simulink model "Mooventure2016_Rev5"  (Simulink 7.7)
settings: Solver=FixedStepDiscrete  StartTime=0.0  StopTime=10  RelTol=1e-3
PreLoadFcn:
  | try, eval([bdroot '_setup']); catch, eval('model_setup', ''); end
InitFcn:
  | try, eval([bdroot '_setup']); catch, eval('model_setup', ''); end
undefined symbols (not defined in the file): ECM, H1, motohawk_build_version, motohawk_trunc_name, motohawk_vardec_config_group, motohawk_vardec_path, xD
libraries: MotoHawk_lib x976, motohawk_control_primitives_lib x41, simulink x27, motohawk_annotations_lib x3
(part 15 of 16)

== system Mooventure2016_Rev5/Foreground/Control/Hybrid Control Code/Cruise Control/Speed Resume ==
  In1 : Inport
  Detect Increase : simulink/Logic and Bit Operations/Detect Increase  SystemSampleTime=-1  vinit=0.0
  Enabled Subsystem1 : Subsystem  TreatAsAtomicUnit=on
  wires:
  In1/1 -> Detect Increase/1
  Detect Increase/1 -> Enabled Subsystem1/Enable

== system Mooventure2016_Rev5/Foreground/Control/Hybrid Control Code/Cruise Control/System Start ==
  In1 : Inport
  Enable : EnablePort
  Constant : Constant  OutDataTypeStr=boolean
  motohawk_data_write : MotoHawk_lib/Data Storage Blocks/motohawk_data_write  source=Lookup By Name  structure=Scalar  operation=Write entire data structure at once  sz_vec=9  sz_row=2  sz_col=9  typ=double  nam='CruiseSpeed'  checkNull=on  write_read_only=off  struct_inst_name=''  struct_name='MyStruct'
  motohawk_data_write1 : MotoHawk_lib/Data Storage Blocks/motohawk_data_write  source=Lookup By Name  structure=Scalar  operation=Write entire data structure at once  sz_vec=9  sz_row=2  sz_col=9  typ=boolean  nam='CruiseOn'  checkNull=on  write_read_only=off  struct_inst_name=''  struct_name='MyStruct'
  wires:
  In1/1 -> motohawk_data_write/1
  Constant/1 -> motohawk_data_write1/1

== system Mooventure2016_Rev5/Foreground/Control/Hybrid Control Code/Hybrid state limits1/Embedded MATLAB Function ==
  ecoMode_Enable : Inport
  SOC : Inport  Port=2
  CHESoC : Inport  Port=3
  SMESoC : Inport  Port=4
  nEV : Inport  Port=5
  Embedded MATLAB Function : Stateflow chart  TreatAsAtomicUnit=on
  state : Outport
  wires:
  ecoMode_Enable/1 -> Embedded MATLAB Function/1(ecoMode_Enable)
  SOC/1 -> Embedded MATLAB Function/2(SOC)
  CHESoC/1 -> Embedded MATLAB Function/3(CHESoC)
  SMESoC/1 -> Embedded MATLAB Function/4(SMESoC)
  nEV/1 -> Embedded MATLAB Function/5(nEV)
  Embedded MATLAB Function/1(state) -> state/1  "state"

== system Mooventure2016_Rev5/Foreground/Control/Hybrid Control Code/IPT/CurrentLimiting_TurboRequest ==
  BatteryCurrent : Inport
  First Order Low Pass (Tunable) : Subsystem  mask(First-Order Low-Pass Filter (Tunable)){nam='Overcurrent_Tq_Lim_Filter', samp_time=-1, group=motohawk_vardec_path(gcb)}
      mask prompts: nam "Name"; samp_time "Sample Time"; group "MotoTune Group String"
      mask help:
      | Discrete first-order low-pass filter, with calibratable time-constant.
      |
      | If 'Sample Time' is -1, then extra code and RAM will be generated to dynamically calculate dt.
      mask Display:
      | patch([0 0 1 1], [0 0.075 0.075 0], [230/255 0/255 0/255])
      | patch([0 0 1 1], [0.025 0.05 0.05 0.025], [150/255 0/255 0/255])
      | patch([0 0 1 1], [0 0.025 0.025 0], [0/255 0/255 0/255])
      | 
      | disp('1st-Order\nLow Pass');
  Gain : Gain  Gain=-1
  OvercurrentIntegralGenerator : Subsystem
  motohawk_probe : MotoHawk_lib/Calibration & Probing Blocks/motohawk_probe  nam='overcurrentintegral_prb'  show_more=off  name_source=Use Parameter  read_level=1  view_as=Number  enum_struct={'Disabled', 'Enabled'}  vector_style=Wide Row  use_help_units=off  help=''  units=''  use_header_enum=off  row_header_enum={}  col_header_enum={}  use_precision=off  precision=''  gain=1  offset=0  exp=1  use_mototune_group=off  mototune_group=motohawk_vardec_path(gcb)
  motohawk_probe1 : MotoHawk_lib/Calibration & Probing Blocks/motohawk_probe  nam='Overcurrent_Torque_Derate_prb'  show_more=off  name_source=Use Parameter  read_level=1  view_as=Number  enum_struct={'Disabled', 'Enabled'}  vector_style=Wide Row  use_help_units=off  help=''  units=''  use_header_enum=off  row_header_enum={}  col_header_enum={}  use_precision=off  precision=''  gain=1  offset=0  exp=1  use_mototune_group=off  mototune_group=motohawk_vardec_path(gcb)
  motohawk_table_1d : MotoHawk_lib/Lookup Tables/motohawk_table_1d  SystemSampleTime=-1  nam='TorqueLimMultiplier'  bp_nam='ModifiedAmpSec'  breakpoint_data=[0,200,900,1500]  table_data=[1,1,0,0]  show_more=off  bp_data_type=Inherit from 'Breakpoint Data'  bp_storage=Constant  table_data_type=Inherit from 'Table Data'  storage=NonAdaptive  read_level=1  write_level=1  ovr_cals=on  use_help=off  help=''  bp_units=''  table_units=''  use_min_max=off  bp_min_val=-inf  bp_max_val=inf  min_val=-inf  max_val=inf  use_precision=off  use_breakpoint=off  b_precision=''  b_gain=1  b_offset=0  b_exp=1  use_table=off  t_precision=''  t_gain=1  t_offset=0  t_exp=1  use_links=off  input_name=''  output_name=''  use_mototune_group=off  mototune_group=motohawk_vardec_path(gcb)
  TorqueMultiplier : Outport
  wires:
  OvercurrentIntegralGenerator/1(OverCurrentIntegral) -> motohawk_table_1d/1, motohawk_probe/1
  BatteryCurrent/1 -> Gain/1
  motohawk_table_1d/1 -> First Order Low Pass (Tunable)/1(in)
  Gain/1 -> OvercurrentIntegralGenerator/1(Current)
  First Order Low Pass (Tunable)/1(out) -> TorqueMultiplier/1, motohawk_probe1/1

== system Mooventure2016_Rev5/Foreground/Control/Hybrid Control Code/IPT/Drive ==
  Enable : EnablePort
  Constant1 : Constant
  motohawk_override_abs4 : MotoHawk_lib/Calibration & Probing Blocks/motohawk_override_abs  SystemSampleTime=-1  parent_name='Torque_Reverse_Override'  parent_val=1  show_more=on  name_source=Use Parameter  parent_read_level=1  parent_override_level=1  view_as=Number  enum_struct={'Disabled', 'Enabled'}  use_help_units=off  parent_help=''  parent_units=''  use_min_max=on  parent_min=-inf  parent_max=inf  use_precision=off  parent_precision=''  parent_gain=1  parent_offset=0  parent_exp=1  use_mototune_group=off  parent_group=motohawk_vardec_path(gcb)
  IPT_Torque : Outport  OutputWhenDisabled=reset  InitialOutput=[0]
  wires:
  Constant1/1 -> motohawk_override_abs4/1
  motohawk_override_abs4/1 -> IPT_Torque/1

== system Mooventure2016_Rev5/Foreground/Control/Hybrid Control Code/IPT/First Order Low Pass (Tunable) ==
  note: Tunable 1st-Order Low-Pass Filter
  in : Inport
  First Order Low Pass : motohawk_control_primitives_lib/First Order Low Pass  SystemSampleTime=-1
  MinMax : MinMax  Function=max  Inputs=2  SaturateOnIntegerOverflow=on  InputSameDT=on
  Product : Product  Inputs=*/  SaturateOnIntegerOverflow=on  InputSameDT=on  OutDataTypeStr=Inherit: Same as first input
  motohawk_calibration : MotoHawk_lib/Calibration & Probing Blocks/motohawk_calibration  nam=nam  val=.4  storage=Calibration  show_more=on  name_source=Use Parameter  data_type=Inherit from 'Default Value'  read_level=1  write_level=1  ovr_cals=on  view_as=Number  enum_struct={'Disabled', 'Enabled'}  vector_style=Wide Row  use_help_units=on  help='Filter time constant'  units='sec'  use_header_enum=off  row_header_enum={}  col_header_enum={}  use_min_max=off  min_val=-inf  max_val=inf  use_precision=off  precision=''  gain=1  offset=0  exp=1  use_mototune_group=on  mototune_group=group %% motohawk_vardec_config_group(group)
  motohawk_delta_time : MotoHawk_lib/Extra Development Blocks/motohawk_delta_time  samp_time=samp_time  init_val=0  mode=Seconds (double)
  out : Outport
  wires:
  First Order Low Pass/1 -> out/1
  in/1 -> First Order Low Pass/1
  motohawk_delta_time/1 -> Product/1, MinMax/1
  Product/1 -> First Order Low Pass/2
  MinMax/1 -> Product/2
  motohawk_calibration/1 -> MinMax/2

== system Mooventure2016_Rev5/Foreground/Control/Hybrid Control Code/IPT/Neutral ==
  Enable : EnablePort
  Constant : Constant  Value=0
  IPT_Torque : Outport
  wires:
  Constant/1 -> IPT_Torque/1  "IPT_Torque"

== system Mooventure2016_Rev5/Foreground/Control/Hybrid Control Code/IPT/Reverse ==
  Enable : EnablePort
  Constant1 : Constant  Value=-1
  motohawk_override_abs4 : MotoHawk_lib/Calibration & Probing Blocks/motohawk_override_abs  SystemSampleTime=-1  parent_name='Torque_Reverse_Override69'  parent_val=1  show_more=on  name_source=Use Parameter  parent_read_level=1  parent_override_level=1  view_as=Number  enum_struct={'Disabled', 'Enabled'}  use_help_units=off  parent_help=''  parent_units=''  use_min_max=on  parent_min=-inf  parent_max=inf  use_precision=off  parent_precision=''  parent_gain=1  parent_offset=0  parent_exp=1  use_mototune_group=off  parent_group=motohawk_vardec_path(gcb)
  IPT_Torque : Outport  OutputWhenDisabled=reset  InitialOutput=[0]
  wires:
  Constant1/1 -> motohawk_override_abs4/1
  motohawk_override_abs4/1 -> IPT_Torque/1

== system Mooventure2016_Rev5/Foreground/Inputs/Analog Inputs/Coolant/Heater Core Low Pass ==
  note: Tunable 1st-Order Low-Pass Filter
  in : Inport
  First Order Low Pass : motohawk_control_primitives_lib/First Order Low Pass  SystemSampleTime=-1
  MinMax : MinMax  Function=max  Inputs=2  SaturateOnIntegerOverflow=on  InputSameDT=on
  Product : Product  Inputs=*/  SaturateOnIntegerOverflow=on  InputSameDT=on  OutDataTypeStr=Inherit: Same as first input
  motohawk_calibration : MotoHawk_lib/Calibration & Probing Blocks/motohawk_calibration  nam=nam  val=.4  storage=Calibration  show_more=on  name_source=Use Parameter  data_type=Inherit from 'Default Value'  read_level=1  write_level=1  ovr_cals=on  view_as=Number  enum_struct={'Disabled', 'Enabled'}  vector_style=Wide Row  use_help_units=on  help='Filter time constant'  units='sec'  use_header_enum=off  row_header_enum={}  col_header_enum={}  use_min_max=off  min_val=-inf  max_val=inf  use_precision=off  precision=''  gain=1  offset=0  exp=1  use_mototune_group=on  mototune_group=group %% motohawk_vardec_config_group(group)
  motohawk_delta_time : MotoHawk_lib/Extra Development Blocks/motohawk_delta_time  samp_time=samp_time  init_val=0  mode=Seconds (double)
  out : Outport
  wires:
  First Order Low Pass/1 -> out/1
  in/1 -> First Order Low Pass/1
  motohawk_delta_time/1 -> Product/1, MinMax/1
  Product/1 -> First Order Low Pass/2
  MinMax/1 -> Product/2
  motohawk_calibration/1 -> MinMax/2

== system Mooventure2016_Rev5/Foreground/Inputs/Analog Inputs/Coolant/Radiator Low Pass ==
  note: Tunable 1st-Order Low-Pass Filter
  in : Inport
  First Order Low Pass : motohawk_control_primitives_lib/First Order Low Pass  SystemSampleTime=-1
  MinMax : MinMax  Function=max  Inputs=2  SaturateOnIntegerOverflow=on  InputSameDT=on
  Product : Product  Inputs=*/  SaturateOnIntegerOverflow=on  InputSameDT=on  OutDataTypeStr=Inherit: Same as first input
  motohawk_calibration : MotoHawk_lib/Calibration & Probing Blocks/motohawk_calibration  nam=nam  val=.4  storage=Calibration  show_more=on  name_source=Use Parameter  data_type=Inherit from 'Default Value'  read_level=1  write_level=1  ovr_cals=on  view_as=Number  enum_struct={'Disabled', 'Enabled'}  vector_style=Wide Row  use_help_units=on  help='Filter time constant'  units='sec'  use_header_enum=off  row_header_enum={}  col_header_enum={}  use_min_max=off  min_val=-inf  max_val=inf  use_precision=off  precision=''  gain=1  offset=0  exp=1  use_mototune_group=on  mototune_group=group %% motohawk_vardec_config_group(group)
  motohawk_delta_time : MotoHawk_lib/Extra Development Blocks/motohawk_delta_time  samp_time=samp_time  init_val=0  mode=Seconds (double)
  out : Outport
  wires:
  First Order Low Pass/1 -> out/1
  in/1 -> First Order Low Pass/1
  motohawk_delta_time/1 -> Product/1, MinMax/1
  Product/1 -> First Order Low Pass/2
  MinMax/1 -> Product/2
  motohawk_calibration/1 -> MinMax/2

== system Mooventure2016_Rev5/Foreground/Inputs/Battery_Inputs/SOC Filter/First Order Low Pass (Tunable) ==
  note: Tunable 1st-Order Low-Pass Filter
  in : Inport
  First Order Low Pass : motohawk_control_primitives_lib/First Order Low Pass  SystemSampleTime=-1
  MinMax : MinMax  Function=max  Inputs=2  SaturateOnIntegerOverflow=on  InputSameDT=on
  Product : Product  Inputs=*/  SaturateOnIntegerOverflow=on  InputSameDT=on  OutDataTypeStr=Inherit: Same as first input
  motohawk_calibration : MotoHawk_lib/Calibration & Probing Blocks/motohawk_calibration  nam=nam  val=5  storage=Calibration  show_more=on  name_source=Use Parameter  data_type=Inherit from 'Default Value'  read_level=1  write_level=1  ovr_cals=on  view_as=Number  enum_struct={'Disabled', 'Enabled'}  vector_style=Wide Row  use_help_units=on  help='Filter time constant'  units='sec'  use_header_enum=off  row_header_enum={}  col_header_enum={}  use_min_max=off  min_val=-inf  max_val=inf  use_precision=off  precision=''  gain=1  offset=0  exp=1  use_mototune_group=on  mototune_group=group %% motohawk_vardec_config_group(group)
  motohawk_delta_time : MotoHawk_lib/Extra Development Blocks/motohawk_delta_time  samp_time=samp_time  init_val=0  mode=Seconds (double)
  out : Outport
  wires:
  First Order Low Pass/1 -> out/1
  in/1 -> First Order Low Pass/1
  motohawk_delta_time/1 -> Product/1, MinMax/1
  Product/1 -> First Order Low Pass/2
  MinMax/1 -> Product/2
  motohawk_calibration/1 -> MinMax/2

== system Mooventure2016_Rev5/Foreground/Inputs/Battery_Inputs/Voltage Filter/First Order Low Pass (Tunable) ==
  note: Tunable 1st-Order Low-Pass Filter
  in : Inport
  First Order Low Pass : motohawk_control_primitives_lib/First Order Low Pass  SystemSampleTime=-1
  MinMax : MinMax  Function=max  Inputs=2  SaturateOnIntegerOverflow=on  InputSameDT=on
  Product : Product  Inputs=*/  SaturateOnIntegerOverflow=on  InputSameDT=on  OutDataTypeStr=Inherit: Same as first input
  motohawk_calibration : MotoHawk_lib/Calibration & Probing Blocks/motohawk_calibration  nam=nam  val=5  storage=Calibration  show_more=on  name_source=Use Parameter  data_type=Inherit from 'Default Value'  read_level=1  write_level=1  ovr_cals=on  view_as=Number  enum_struct={'Disabled', 'Enabled'}  vector_style=Wide Row  use_help_units=on  help='Filter time constant'  units='sec'  use_header_enum=off  row_header_enum={}  col_header_enum={}  use_min_max=off  min_val=-inf  max_val=inf  use_precision=off  precision=''  gain=1  offset=0  exp=1  use_mototune_group=on  mototune_group=group %% motohawk_vardec_config_group(group)
  motohawk_delta_time : MotoHawk_lib/Extra Development Blocks/motohawk_delta_time  samp_time=samp_time  init_val=0  mode=Seconds (double)
  out : Outport
  wires:
  First Order Low Pass/1 -> out/1
  in/1 -> First Order Low Pass/1
  motohawk_delta_time/1 -> Product/1, MinMax/1
  Product/1 -> First Order Low Pass/2
  MinMax/1 -> Product/2
  motohawk_calibration/1 -> MinMax/2

== system Mooventure2016_Rev5/Foreground/Control/Faults/Accesories/HV-Heater System/Triggered Subsystem ==
  In1 : Inport
  Trigger : TriggerPort
  motohawk_data_write : MotoHawk_lib/Data Storage Blocks/motohawk_data_write  source=Lookup By Name  structure=Scalar  operation=Write entire data structure at once  sz_vec=9  sz_row=2  sz_col=9  typ=double  nam='TempReading'  checkNull=on  write_read_only=off  struct_inst_name=''  struct_name='MyStruct'
  wires:
  In1/1 -> motohawk_data_write/1

== system Mooventure2016_Rev5/Foreground/Control/Hybrid Control Code/Cruise Control/Speed Changing/Speed Decrease ==
  Enable : EnablePort
  Add : Sum  Inputs=+-
  Constant : Constant
  motohawk_data_read1 : MotoHawk_lib/Data Storage Blocks/motohawk_data_read  source=Lookup By Name  structure=Scalar  operation=Read scalar from location by index  sz_vec=4  sz_row=2  sz_col=3  typ=double  nam='CruiseSpeed'  checkNull=on  struct_inst_name='MyData'  struct_nam='MyStruct'
  motohawk_data_write : MotoHawk_lib/Data Storage Blocks/motohawk_data_write  source=Lookup By Name  structure=Scalar  operation=Write entire data structure at once  sz_vec=9  sz_row=2  sz_col=9  typ=double  nam='CruiseSpeed'  checkNull=on  write_read_only=off  struct_inst_name=''  struct_name='MyStruct'
  wires:
  motohawk_data_read1/1 -> Add/1
  Constant/1 -> Add/2
  Add/1 -> motohawk_data_write/1

== system Mooventure2016_Rev5/Foreground/Control/Hybrid Control Code/Cruise Control/Speed Changing/Speed Increase ==
  Enable : EnablePort
  Add : Sum
  Constant : Constant
  motohawk_data_read1 : MotoHawk_lib/Data Storage Blocks/motohawk_data_read  source=Lookup By Name  structure=Scalar  operation=Read scalar from location by index  sz_vec=4  sz_row=2  sz_col=3  typ=double  nam='CruiseSpeed'  checkNull=on  struct_inst_name='MyData'  struct_nam='MyStruct'
  motohawk_data_write : MotoHawk_lib/Data Storage Blocks/motohawk_data_write  source=Lookup By Name  structure=Scalar  operation=Write entire data structure at once  sz_vec=9  sz_row=2  sz_col=9  typ=double  nam='CruiseSpeed'  checkNull=on  write_read_only=off  struct_inst_name=''  struct_name='MyStruct'
  wires:
  motohawk_data_read1/1 -> Add/1
  Constant/1 -> Add/2
  Add/1 -> motohawk_data_write/1

== system Mooventure2016_Rev5/Foreground/Control/Hybrid Control Code/Cruise Control/Speed Control/PID With Damper Terms (Tunable) ==
  note: PID With Damper Terms
      | With Calibratable Parameters and Observable States
  Actual : Inport
  SetPoint : Inport  Port=2
  ResetITerm : Inport  Port=3
  Ground2 : Ground
  PID With Damper Terms : Subsystem  Description=|  AncestorBlock=motohawk_control_primitives_lib/PID With Damper Terms  mask(PID with Damper Terms){samp_time=SampleTime}
      | /* Name: ErrorGain Unit:mult ClassID:VAR StorageID:FLASH Access:RW4+RW3+NA2+NA1 TypeID:UINT4                   
      |    Gain:0.000000001 Min:0.000000000 Max:4.000000000 Format:10.9 UpdateID:REMOTE Help:"This gain is applied to "
      |    "the error term before it is used to calculate the P, I and D terms." VardecSig:6C */                       
      |                                                                                                                
      | /* Name: ITermLowerLim Unit:0 ClassID:VAR StorageID:FLASH Access:RW4+RW3+NA2+NA1 TypeID:SINT2 Gain:0.1         
      |    Min:-3276.8 Max:3276.7 Format:5.1 UpdateID:REMOTE Help:"Lower limit on the I-term value." VardecSig:6C */   
      |                                                                                                                
      | /* Name: ITermUpperLim ClassID:VAR StorageID:FLASH Access:RW4+RW3+NA2+NA1 TypeID:SINT2 Gain:0.1 Min:-3276.8    
      |    Max:3276.7 Format:5.1 UpdateID:REMOTE Help:"Upper limit on I-term value." VardecSig:6C */                   
      |                                                                                                                
      | /* Name: PIDOutLowerLim ClassID:VAR StorageID:FLASH Access:RW4+RW3+NA2+NA1 TypeID:SINT2 Gain:0.1               
      |    Min:-3276.8 Max:3276.7 Format:5.1 UpdateID:REMOTE Help:"Lower limit on PID output." VardecSig:6C */         
      |                                                                                                                
      | /* Name: PIDOutUpperLim ClassID:VAR StorageID:FLASH Access:RW4+RW3+NA2+NA1 TypeID:SINT2 Gain:0.1               
      |    Min:-3276.8 Max:3276.7 Format:3.1 UpdateID:REMOTE Help:"Upper limit on PID output." VardecSig:6C */         
      |                                                                                                                
      | /* Name: PIDError ClassID:VAR StorageID:RAM Access:RO4+RO3+NA2+NA1 TypeID:SINT2 Gain:1 Min:-32768.00           
      |    Max:32767.00 Format:4.2 UpdateID:BACKGND Help:"Current controller error input value." VardecSig:6C */       
      |                                                                                                                
      | /* Name: PTerm ClassID:VAR StorageID:RAM Access:RO4+RO3+NA2+NA1 TypeID:SINT2 Gain:1 Min:-32768.00              
      |    Max:32767.00 Format:4.2 UpdateID:BACKGND Help:"Current P-term value" VardecSig:6C */                        
      |                                                                                                                
      | /* Name: ITerm ClassID:VAR StorageID:RAM Access:RO4+RO3+NA2+NA1 TypeID:SINT2 Gain:1 Min:-32768.00              
      |    Max:32767.00 Format:4.2 UpdateID:BACKGND Help:"Current I-term value" VardecSig:6C */                        
      |                                                                                                                
      | /* Name: DTerm ClassID:VAR StorageID:RAM Access:RO4+RO3+NA2+NA1 TypeID:SINT2 Gain:1 Min:-32768.00              
      |    Max:32767.00 Format:4.2 UpdateID:BACKGND Help:"Current D-term value" VardecSig:6C */                        
      |                                                                                                                
      | /* Name: DamperTerm ClassID:VAR StorageID:RAM Access:RO4+RO3+NA2+NA1 TypeID:SINT2 Gain:1 Min:-32768.00         
      |    Max:32767.00 Format:4.2 UpdateID:BACKGND Help:"Current Damper-term value" VardecSig:6C */                   
      |                                                                                                                
      | /* Name: PIDOutput ClassID:VAR StorageID:FLASH Access:RW4+RW3+NA2+NA1 TypeID:SINT2 Gain:1 Min:-32768.00        
      |    Max:32767.00 Format:4.2 UpdateID:REMOTE Help:"PID current output." VardecSig:6C */
      mask prompts: samp_time "Sample Time"
      mask help:
      | Resettable PID controller with damper terms and limits on the I-term.
      |
      | If 'Sample Time' is -1, then extra code and RAM will be generated to dynamically calculate dt.
      mask Display:
      | patch([0 0 1 1], 0.5*[0 0.075 0.075 0], [230/255 0/255 0/255])
      | patch([0 0 1 1], 0.5*[0.025 0.05 0.05 0.025], [150/255 0/255 0/255])
      | patch([0 0 1 1], 0.5*[0 0.025 0.025 0], [0/255 0/255 0/255])
      | 
      | disp('\fontsize{16}\bf\itPIDD', 'texmode', 'on')
  Saturation (Tunable) : motohawk_control_primitives_lib/Saturation (Tunable)  SystemSampleTime=-1  prefix=prefix  units=units  grp=grp
  Sum : Sum  Inputs=++|  InputSameDT=on
  motohawk_calibration : MotoHawk_lib/Calibration & Probing Blocks/motohawk_calibration  nam=[prefix 'PGain']  val=1  storage=Calibration  show_more=on  name_source=Use Parameter  data_type=Inherit from 'Default Value'  read_level=1  write_level=1  ovr_cals=on  view_as=Number  enum_struct={'Disabled', 'Enabled'}  vector_style=Wide Row  use_help_units=on  help='PID Proportional Gain'  units='mult'  use_header_enum=off  row_header_enum={}  col_header_enum={}  use_min_max=off  min_val=-inf  max_val=inf  use_precision=off  precision=''  gain=1  offset=0  exp=1  use_mototune_group=on  mototune_group=grp
  motohawk_calibration1 : MotoHawk_lib/Calibration & Probing Blocks/motohawk_calibration  nam=[prefix 'DGain']  val=1  storage=Calibration  show_more=on  name_source=Use Parameter  data_type=Inherit from 'Default Value'  read_level=1  write_level=1  ovr_cals=on  view_as=Number  enum_struct={'Disabled', 'Enabled'}  vector_style=Wide Row  use_help_units=on  help='PID Derivative Gain'  units='mult'  use_header_enum=off  row_header_enum={}  col_header_enum={}  use_min_max=off  min_val=-inf  max_val=inf  use_precision=off  precision=''  gain=1  offset=0  exp=1  use_mototune_group=on  mototune_group=grp
  motohawk_calibration2 : MotoHawk_lib/Calibration & Probing Blocks/motohawk_calibration  nam=[prefix 'IGain']  val=1  storage=Calibration  show_more=on  name_source=Use Parameter  data_type=Inherit from 'Default Value'  read_level=1  write_level=1  ovr_cals=on  view_as=Number  enum_struct={'Disabled', 'Enabled'}  vector_style=Wide Row  use_help_units=on  help='PID Integral Gain'  units='mult'  use_header_enum=off  row_header_enum={}  col_header_enum={}  use_min_max=off  min_val=-inf  max_val=inf  use_precision=off  precision=''  gain=1  offset=0  exp=1  use_mototune_group=on  mototune_group=grp
  motohawk_calibration3 : MotoHawk_lib/Calibration & Probing Blocks/motohawk_calibration  nam=[prefix 'IMin']  val=0  storage=Calibration  show_more=on  name_source=Use Parameter  data_type=Inherit from 'Default Value'  read_level=1  write_level=1  ovr_cals=on  view_as=Number  enum_struct={'Disabled', 'Enabled'}  vector_style=Wide Row  use_help_units=on  help='PID Integrator Lower Limit'  units=units  use_header_enum=off  row_header_enum={}  col_header_enum={}  use_min_max=off  min_val=-inf  max_val=inf  use_precision=off  precision=''  gain=1  offset=0  exp=1  use_mototune_group=on  mototune_group=grp
  motohawk_calibration4 : MotoHawk_lib/Calibration & Probing Blocks/motohawk_calibration  nam=[prefix 'IMax']  val=1  storage=Calibration  show_more=on  name_source=Use Parameter  data_type=Inherit from 'Default Value'  read_level=1  write_level=1  ovr_cals=on  view_as=Number  enum_struct={'Disabled', 'Enabled'}  vector_style=Wide Row  use_help_units=on  help='PID Integrator Upper Limit'  units=units  use_header_enum=off  row_header_enum={}  col_header_enum={}  use_min_max=off  min_val=-inf  max_val=inf  use_precision=off  precision=''  gain=1  offset=0  exp=1  use_mototune_group=on  mototune_group=grp
  motohawk_calibration5 : MotoHawk_lib/Calibration & Probing Blocks/motohawk_calibration  nam=[prefix 'DCOffset']  val=0  storage=Calibration  show_more=on  name_source=Use Parameter  data_type=Inherit from 'Default Value'  read_level=1  write_level=1  ovr_cals=on  view_as=Number  enum_struct={'Disabled', 'Enabled'}  vector_style=Wide Row  use_help_units=on  help='PID Output DC Offset'  units=units  use_header_enum=off  row_header_enum={}  col_header_enum={}  use_min_max=off  min_val=-inf  max_val=inf  use_precision=off  precision=''  gain=1  offset=0  exp=1  use_mototune_group=on  mototune_group=grp
  motohawk_calibration6 : MotoHawk_lib/Calibration & Probing Blocks/motohawk_calibration  nam=[prefix 'ErrorGain']  val=1  storage=Calibration  show_more=on  name_source=Use Parameter  data_type=Inherit from 'Default Value'  read_level=1  write_level=1  ovr_cals=on  view_as=Number  enum_struct={'Disabled', 'Enabled'}  vector_style=Wide Row  use_help_units=on  help='PID Error Gain'  units='mult'  use_header_enum=off  row_header_enum={}  col_header_enum={}  use_min_max=off  min_val=-inf  max_val=inf  use_precision=off  precision=''  gain=1  offset=0  exp=1  use_mototune_group=on  mototune_group=grp
  motohawk_calibration7 : MotoHawk_lib/Calibration & Probing Blocks/motohawk_calibration  nam=[prefix 'DampGainUp']  val=1  storage=Calibration  show_more=on  name_source=Use Parameter  data_type=Inherit from 'Default Value'  read_level=1  write_level=1  ovr_cals=on  view_as=Number  enum_struct={'Disabled', 'Enabled'}  vector_style=Wide Row  use_help_units=on  help='PID Damper Gain - Up Direction'  units='mult'  use_header_enum=off  row_header_enum={}  col_header_enum={}  use_min_max=off  min_val=-inf  max_val=inf  use_precision=off  precision=''  gain=1  offset=0  exp=1  use_mototune_group=on  mototune_group=grp
  motohawk_calibration8 : MotoHawk_lib/Calibration & Probing Blocks/motohawk_calibration  nam=[prefix 'DampGainDown']  val=1  storage=Calibration  show_more=on  name_source=Use Parameter  data_type=Inherit from 'Default Value'  read_level=1  write_level=1  ovr_cals=on  view_as=Number  enum_struct={'Disabled', 'Enabled'}  vector_style=Wide Row  use_help_units=on  help='PID Damper Gain - Down Direction'  units='mult'  use_header_enum=off  row_header_enum={}  col_header_enum={}  use_min_max=off  min_val=-inf  max_val=inf  use_precision=off  precision=''  gain=1  offset=0  exp=1  use_mototune_group=on  mototune_group=grp
  motohawk_probe : MotoHawk_lib/Calibration & Probing Blocks/motohawk_probe  nam=[prefix 'Out']  show_more=on  name_source=Use Parameter  read_level=1  view_as=Number  enum_struct={'Disabled', 'Enabled'}  vector_style=Wide Row  use_help_units=on  help='PID Final Output'  units=units  use_header_enum=off  row_header_enum={}  col_header_enum={}  use_precision=off  precision=''  gain=1  offset=0  exp=1  use_mototune_group=on  mototune_group=grp
  motohawk_probe1 : MotoHawk_lib/Calibration & Probing Blocks/motohawk_probe  nam=[prefix 'PTerm']  show_more=on  name_source=Use Parameter  read_level=1  view_as=Number  enum_struct={'Disabled', 'Enabled'}  vector_style=Wide Row  use_help_units=on  help='PID Proportional Term'  units=units  use_header_enum=off  row_header_enum={}  col_header_enum={}  use_precision=off  precision=''  gain=1  offset=0  exp=1  use_mototune_group=on  mototune_group=grp
  motohawk_probe2 : MotoHawk_lib/Calibration & Probing Blocks/motohawk_probe  nam=[prefix 'ITerm']  show_more=on  name_source=Use Parameter  read_level=1  view_as=Number  enum_struct={'Disabled', 'Enabled'}  vector_style=Wide Row  use_help_units=on  help='PID Integrator Term'  units=units  use_header_enum=off  row_header_enum={}  col_header_enum={}  use_precision=off  precision=''  gain=1  offset=0  exp=1  use_mototune_group=on  mototune_group=grp
  motohawk_probe3 : MotoHawk_lib/Calibration & Probing Blocks/motohawk_probe  nam=[prefix 'DTerm']  show_more=on  name_source=Use Parameter  read_level=1  view_as=Number  enum_struct={'Disabled', 'Enabled'}  vector_style=Wide Row  use_help_units=on  help='PID Derivative Term'  units=units  use_header_enum=off  row_header_enum={}  col_header_enum={}  use_precision=off  precision=''  gain=1  offset=0  exp=1  use_mototune_group=on  mototune_group=grp
  motohawk_probe4 : MotoHawk_lib/Calibration & Probing Blocks/motohawk_probe  nam=[prefix 'Error']  show_more=on  name_source=Use Parameter  read_level=1  view_as=Number  enum_struct={'Disabled', 'Enabled'}  vector_style=Wide Row  use_help_units=on  help='PID Error Term'  units=units  use_header_enum=off  row_header_enum={}  col_header_enum={}  use_precision=off  precision=''  gain=1  offset=0  exp=1  use_mototune_group=on  mototune_group=grp
  motohawk_probe5 : MotoHawk_lib/Calibration & Probing Blocks/motohawk_probe  nam=[prefix 'DampTerm']  show_more=on  name_source=Use Parameter  read_level=1  view_as=Number  enum_struct={'Disabled', 'Enabled'}  vector_style=Wide Row  use_help_units=on  help='PID Damper Term'  units=units  use_header_enum=off  row_header_enum={}  col_header_enum={}  use_precision=off  precision=''  gain=1  offset=0  exp=1  use_mototune_group=on  mototune_group=grp
  Out : Outport
  wires:
  motohawk_calibration5/1 -> Sum/1
  Sum/1 -> Saturation (Tunable)/1
  ResetITerm/1 -> PID With Damper Terms/12(I_reset)
  Ground2/1 -> PID With Damper Terms/9(IC)
  motohawk_calibration1/1 -> PID With Damper Terms/6(k_D)
  motohawk_calibration2/1 -> PID With Damper Terms/5(k_I)
  motohawk_calibration/1 -> PID With Damper Terms/4(k_P)
  PID With Damper Terms/3(P_term) -> motohawk_probe1/1
  Actual/1 -> PID With Damper Terms/1(Actual)
  SetPoint/1 -> PID With Damper Terms/2(SetPt)
  PID With Damper Terms/1(Out) -> Sum/2
  motohawk_calibration6/1 -> PID With Damper Terms/3(k_Err)
  motohawk_calibration3/1 -> PID With Damper Terms/10(I_min)
  motohawk_calibration4/1 -> PID With Damper Terms/11(I_max)
  PID With Damper Terms/4(I_term) -> motohawk_probe2/1
  PID With Damper Terms/5(D_term) -> motohawk_probe3/1
  PID With Damper Terms/2(Err) -> motohawk_probe4/1
  motohawk_calibration7/1 -> PID With Damper Terms/7(k_Dmp,u)
  motohawk_calibration8/1 -> PID With Damper Terms/8(k_Dmp,d)
  PID With Damper Terms/6(Dmp_term) -> motohawk_probe5/1
  Saturation (Tunable)/1 -> Out/1, motohawk_probe/1

== system Mooventure2016_Rev5/Foreground/Control/Hybrid Control Code/Cruise Control/Speed Resume/Enabled Subsystem1 ==
  Enable : EnablePort
  Constant : Constant  OutDataTypeStr=boolean
  motohawk_data_write1 : MotoHawk_lib/Data Storage Blocks/motohawk_data_write  source=Lookup By Name  structure=Scalar  operation=Write entire data structure at once  sz_vec=9  sz_row=2  sz_col=9  typ=boolean  nam='CruiseOn'  checkNull=on  write_read_only=off  struct_inst_name=''  struct_name='MyStruct'
  wires:
  Constant/1 -> motohawk_data_write1/1

== system Mooventure2016_Rev5/Foreground/Control/Hybrid Control Code/IPT/CurrentLimiting_TurboRequest/First Order Low Pass (Tunable) ==
  note: Tunable 1st-Order Low-Pass Filter
  in : Inport
  First Order Low Pass : motohawk_control_primitives_lib/First Order Low Pass  SystemSampleTime=-1
  MinMax : MinMax  Function=max  Inputs=2  SaturateOnIntegerOverflow=on  InputSameDT=on
  Product : Product  Inputs=*/  SaturateOnIntegerOverflow=on  InputSameDT=on  OutDataTypeStr=Inherit: Same as first input
  motohawk_calibration : MotoHawk_lib/Calibration & Probing Blocks/motohawk_calibration  nam=nam  val=.005  storage=Calibration  show_more=on  name_source=Use Parameter  data_type=Inherit from 'Default Value'  read_level=1  write_level=1  ovr_cals=on  view_as=Number  enum_struct={'Disabled', 'Enabled'}  vector_style=Wide Row  use_help_units=on  help='Filter time constant'  units='sec'  use_header_enum=off  row_header_enum={}  col_header_enum={}  use_min_max=off  min_val=-inf  max_val=inf  use_precision=off  precision=''  gain=1  offset=0  exp=1  use_mototune_group=on  mototune_group=group %% motohawk_vardec_config_group(group)
  motohawk_delta_time : MotoHawk_lib/Extra Development Blocks/motohawk_delta_time  samp_time=samp_time  init_val=0  mode=Seconds (double)
  out : Outport
  wires:
  First Order Low Pass/1 -> out/1
  in/1 -> First Order Low Pass/1
  motohawk_delta_time/1 -> Product/1, MinMax/1
  Product/1 -> First Order Low Pass/2
  MinMax/1 -> Product/2
  motohawk_calibration/1 -> MinMax/2

== system Mooventure2016_Rev5/Foreground/Control/Hybrid Control Code/IPT/CurrentLimiting_TurboRequest/OvercurrentIntegralGenerator ==
  note: max over current integral allowed
  Current : Inport
  Constant : Constant  Value=0
  Constant1 : Constant  Value=1500
  Constant2 : Constant  Value=0
  Constant3 : Constant  Value=0
  CurrentModifier : Subsystem
  Integrator : Subsystem  mask(Discrete Integrator){samp_time=-1}
      mask prompts: samp_time "Sample Time"
      mask help:
      | Resetable integrator with upper and lower windup limits.
      |
      | If 'Sample Time' is -1, then extra code and RAM will be generated to dynamically calculate dt.
      mask Display:
      | patch([0 0 1 1], 0.75*[0 0.075 0.075 0], [230/255 0/255 0/255])
      | patch([0 0 1 1], 0.75*[0.025 0.05 0.05 0.025], [150/255 0/255 0/255])
      | patch([0 0 1 1], 0.75*[0 0.025 0.025 0], [0/255 0/255 0/255])
      | 
      | disp('\fontsize{16}\bf\it\int dt', 'texmode', 'on')
  OverCurrentIntegral : Outport
  wires:
  Constant2/1 -> Integrator/3(IC)
  Constant/1 -> Integrator/4(Min)
  Constant1/1 -> Integrator/5(Max)
  Constant3/1 -> Integrator/2(Rst)
  CurrentModifier/1(Out1) -> Integrator/1(In)
  Current/1 -> CurrentModifier/1(In1)
  Integrator/1(Out) -> OverCurrentIntegral/1

== system Mooventure2016_Rev5/Foreground/Control/Hybrid Control Code/Cruise Control/Speed Control/PID With Damper Terms (Tunable)/PID With Damper Terms ==
  note: Universal PID Controller
      | with Dampers
  Actual : Inport
  SetPt : Inport  Port=2
  k_Err : Inport  Port=3
  k_P : Inport  Port=4
  k_I : Inport  Port=5
  k_D : Inport  Port=6
  k_Dmp,u : Inport  Port=7
  k_Dmp,d : Inport  Port=8
  IC : Inport  Port=9
  I_min : Inport  Port=10
  I_max : Inport  Port=11
  I_reset : Inport  Port=12
  Constant : Constant  Value=0  OutDataTypeStr=Inherit: Inherit via back propagation
  Data Type Conversion : DataTypeConversion  SaturateOnIntegerOverflow=on  RndMeth=Zero
  Derivitive1 : motohawk_control_primitives_lib/Derivitive  SystemSampleTime=-1  samp_time=samp_time
  Derivitive2 : motohawk_control_primitives_lib/Derivitive  SystemSampleTime=-1  samp_time=samp_time
  Derivitive3 : motohawk_control_primitives_lib/Derivitive  SystemSampleTime=-1  samp_time=samp_time
  Integrator : motohawk_control_primitives_lib/Integrator  SystemSampleTime=-1  samp_time=samp_time
  Product{1..5} (5 alike) : Product  InputSameDT=on  OutDataTypeStr=Inherit: Same as first input
  Relational Operator : RelationalOperator  Operator=>  ZeroCross=off  InputSameDT=on
  Sum : Sum  Inputs=-|+|+|+  SaturateOnIntegerOverflow=on  InputSameDT=on  OutDataTypeStr=Inherit: Same as first input
  Sum2 : Sum  Inputs=-|+  SaturateOnIntegerOverflow=on  InputSameDT=on  OutDataTypeStr=Inherit: Same as first input
  Switch : Switch  Threshold=1  ZeroCross=off  InputSameDT=on
  Out : Outport
  Err : Outport  Port=2
  P_term : Outport  Port=3
  I_term : Outport  Port=4
  D_term : Outport  Port=5
  Dmp_term : Outport  Port=6
  wires:
  Derivitive1/1 -> Sum/1, Dmp_term/1
  Derivitive3/1 -> Sum/2, D_term/1
  Product4/1 -> Derivitive3/1
  k_D/1 -> Product4/1
  SetPt/1 -> Sum2/2
  Sum2/1 -> Data Type Conversion/1
  Product5/1 -> Product4/2, Product2/2, Product1/1
  IC/1 -> Integrator/3
  Sum/1 -> Out/1
  Integrator/1 -> Sum/4, I_term/1
  Product2/1 -> Sum/3, P_term/1
  Product1/1 -> Integrator/1
  k_I/1 -> Product1/2
  k_P/1 -> Product2/1
  Actual/1 -> Product3/2, Derivitive2/1, Sum2/1
  I_reset/1 -> Integrator/2
  k_Err/1 -> Product5/2
  Data Type Conversion/1 -> Err/1, Product5/1
  I_min/1 -> Integrator/4
  I_max/1 -> Integrator/5
  Constant/1 -> Relational Operator/2
  Relational Operator/1 -> Switch/2
  Derivitive2/1 -> Relational Operator/1
  Switch/1 -> Product3/1
  k_Dmp,d/1 -> Switch/3
  k_Dmp,u/1 -> Switch/1
  Product3/1 -> Derivitive1/1

== system Mooventure2016_Rev5/Foreground/Control/Hybrid Control Code/IPT/CurrentLimiting_TurboRequest/OvercurrentIntegralGenerator/CurrentModifier ==
  note: current > 160, i^(3.172)
      | 125 < current < 160, i*0.0197 + 0.1003
      | current < 125, torquerecoveryvalue
  In1 : Inport
  Compare To Zero : simulink/Logic and Bit Operations/Compare To Zero  SystemSampleTime=-1  relop=>=  LogicOutDataTypeMode=uint8
  Divide : Product  Inputs=*/
  LimitingBegins : Constant  Value=125
  LimitingBegins1 : Constant  Value=100000
  LimitingBegins2 : Constant  Value=3.172
  Math Function : Math  Operator=pow  SaturateOnIntegerOverflow=on
  Product : Product  RndMeth=Zero
  Relational Operator : RelationalOperator  Operator=>  OutDataTypeStr=boolean
  Sum : Sum  Inputs=|+-
  Sum1 : Sum  Inputs=|++
  Switch : Switch  Criteria=u2 ~= 0
  Switch1 : Switch  Criteria=u2 ~= 0
  exponentiallimt : Constant  Value=160
  motohawk_calibration : MotoHawk_lib/Calibration & Probing Blocks/motohawk_calibration  nam='TorqueRecoveryValue'  val=-5  storage=Calibration  show_more=on  name_source=Use Parameter  data_type=Inherit from 'Default Value'  read_level=1  write_level=1  ovr_cals=on  view_as=Number  enum_struct={'Disabled', 'Enabled'}  vector_style=Wide Row  use_help_units=on  help='Determines indirectly rate/sec at which torque recovers. More negative faster recovery'  units='ModifiedAmps'  use_header_enum=off  row_header_enum={}  col_header_enum={}  use_min_max=off  min_val=-inf  max_val=inf  use_precision=off  precision=''  gain=1  offset=0  exp=1  use_mototune_group=off  mototune_group=motohawk_vardec_path(gcb)
  slope : Constant  Value=0.0197
  yintercept : Constant  Value=0.1003
  Out1 : Outport
  wires:
  LimitingBegins2/1 -> Math Function/2
  Math Function/1 -> Divide/1
  LimitingBegins1/1 -> Divide/2
  Divide/1 -> Switch/3
  LimitingBegins/1 -> Sum/2
  Sum/1 -> Math Function/1, Product/2, Compare To Zero/1
  In1/1 -> Sum/1, Relational Operator/2
  exponentiallimt/1 -> Relational Operator/1
  Relational Operator/1 -> Switch/2
  slope/1 -> Product/1
  Product/1 -> Sum1/2
  yintercept/1 -> Sum1/1
  Sum1/1 -> Switch/1
  Switch/1 -> Switch1/1
  Switch1/1 -> Out1/1
  Compare To Zero/1 -> Switch1/2
  motohawk_calibration/1 -> Switch1/3

== system Mooventure2016_Rev5/Foreground/Control/Hybrid Control Code/IPT/CurrentLimiting_TurboRequest/OvercurrentIntegralGenerator/Integrator ==
  note: Discrete Integrator,
      | with output and state saturation.
  In : Inport
  Rst : Inport  Port=2
  IC : Inport  Port=3
  Min : Inport  Port=4
  Max : Inport  Port=5
  Data Type Conversion : DataTypeConversion  OutDataTypeStr=boolean  RndMeth=Zero
  Product : Product  SaturateOnIntegerOverflow=on  InputSameDT=on  OutDataTypeStr=Inherit: Same as first input
  Saturation : motohawk_control_primitives_lib/Saturation  SystemSampleTime=-1
  Sum : Sum  Inputs=++|  SaturateOnIntegerOverflow=on  InputSameDT=on
  Switch1 : Switch  Threshold=1  ZeroCross=off  SaturateOnIntegerOverflow=on  InputSameDT=on
  Unit Delay : UnitDelay  SampleTime=-1
  motohawk_delta_time : MotoHawk_lib/Extra Development Blocks/motohawk_delta_time  samp_time=-1  init_val=0  mode=Seconds (double)
  Out : Outport
  wires:
  IC/1 -> Switch1/1
  Max/1 -> Saturation/3
  Min/1 -> Saturation/2
  Data Type Conversion/1 -> Switch1/2
  Rst/1 -> Data Type Conversion/1
  Unit Delay/1 -> Switch1/3
  Product/1 -> Sum/2
  In/1 -> Product/1
  motohawk_delta_time/1 -> Product/2
  Switch1/1 -> Sum/1, Out/1
  Sum/1 -> Saturation/1
  Saturation/1 -> Unit Delay/1

== stateflow chart Foreground/Control/Vehicle Run/Stop Determination/Chart ==
  state Initial
    during:
    Vehicle_Enable=false
    Vehicle_Ready=false
    Torque_Enable=false
    Keyed_Relay=true;
  state Batterybootup
    during:
    Vehicle_Enable=true
    Vehicle_Ready=false
    Torque_Enable=false
    Keyed_Relay=true;
  state Charging_and_Temp
    during:
    Vehicle_Enable=true
    Vehicle_Ready=true
    Torque_Enable=false
    Keyed_Relay=true;
  state Normal_Operation
    during:
    Vehicle_Enable=true
    Vehicle_Ready=true
    Torque_Enable=true
    Keyed_Relay=true;
  state Shutdown_Sequence
    during:
    Vehicle_Enable=false
    Vehicle_Ready=false
    Torque_Enable=false
    Keyed_Relay=true;
  state Kill_Component_Keyed
    during:
    Vehicle_Enable=false
    Vehicle_Ready=false
    Torque_Enable=false
    Keyed_Relay=false;
  state Counting
    en: count=0;
    du: count++;
  (default) -> Initial
  Initial -> Batterybootup [order 1] : [!Shutdown]
  Initial -> Shutdown_Sequence [order 2] : [Shutdown]
  Charging_and_Temp -> Normal_Operation [order 1] : [!Charging]
  Batterybootup -> Shutdown_Sequence [order 1] : [Shutdown]
  Shutdown_Sequence -> Kill_Component_Keyed : [!Batt_Contactor_Status]
  Batterybootup -> Charging_and_Temp [order 2] : [Batt_Load_Enable]
  Normal_Operation -> Charging_and_Temp [order 1] : [Charging]
  Counting -> Shutdown_Sequence [order 1] : [count>=200]
  Counting -> Normal_Operation [order 2] : [!Shutdown]
  Charging_and_Temp -> Counting [order 2] : [Shutdown]
  Normal_Operation -> Counting [order 2] : [Shutdown]
  data: Shutdown input boolean; Batt_Load_Enable input boolean; Vehicle_Enable output boolean; Vehicle_Ready output boolean; Torque_Enable output boolean; Keyed_Relay output boolean; Batt_Contactor_Status input boolean; Charging input boolean; count local double

== matlab function Foreground/Control/Hybrid Control Code/Hybrid state limits1/Embedded MATLAB Function/Embedded MATLAB Function ==
  data: ecoMode_Enable input double; state output double; SOC input double; CHESoC input double; SMESoC input double; nEV input double
function state = fcn(ecoMode_Enable, SOC, CHESoC, SMESoC, nEV)
    if(nEV || (SOC <= SMESoC))
        state = 0;
    elseif ((SOC > SMESoC)&&(SOC <= CHESoC))
        state = 1;
    elseif((ecoMode_Enable == 1)&&(SOC > CHESoC))
        state = 2;
    else
        state = 3;
    end

== matlab function Foreground/Inputs/Driver Inputs/Embedded MATLAB Function1 ==
  data: driver1 input double; driverTemp output double; driver10 input double
function driverTemp = fcn(driver1,driver10)

driverTemp = driver10 * 10 + driver1;

== stateflow chart Foreground/Outputs/IPT Outputs/OnOff Delay ==
  state MotorDisabled
    entry: motorcount=0;
    during: MotorEnable=0;
    during: IPTWake=1;
    during: IPTEnable=1;
  state MotorEnabled
    entry: motorcount=0;
    during: MotorEnable=1;
    during: IPTWake=1;
    during: IPTEnable=1;
  state TimerRunningOne
    during: motorcount++;
  state TimerRunningTwo
    during: motorcount++;
  state Init
    during: MotorEnable=0;
    during: IPTWake=0;
    during: IPTEnable=0;
  state IPTAwake
    during: IPTWake=1;
    during: IPTEnable=0;
    during: MotorEnable=0;
  state IPTEnable
    during: IPTWake=1;
    during: IPTEnable=1;
    during: MotorEnable=0;
  TimerRunningTwo -> MotorDisabled [order 2] : [motorcount>=Motor_Kill_Time]
  MotorDisabled -> TimerRunningOne : [MotorReady]
  TimerRunningOne -> MotorEnabled [order 1] : [motorcount>=Motor_Kill_Time]
  TimerRunningOne -> MotorDisabled [order 2] : [~MotorReady]
  MotorEnabled -> TimerRunningTwo : [~MotorReady]
  TimerRunningTwo -> MotorEnabled [order 1] : [MotorReady]
  (default) -> Init
  Init -> IPTAwake : [VehicleReady && after(1,sec)]
  IPTAwake -> IPTEnable : [after(0.5,sec)]
  IPTEnable -> MotorDisabled : [MotorReady && after(1,sec)]
  data: MotorReady input boolean; MotorEnable output boolean; motorcount local int32; Motor_Kill_Time input int32; IPTWake output boolean; IPTEnable output boolean; VehicleReady input boolean

== matlab function Foreground/Inputs/Driver Inputs/Embedded MATLAB Function2 ==
  data: passenger1 input double; passengerTemp output double; passenger10 input double
function passengerTemp = fcn(passenger1,passenger10)

passengerTemp = passenger10 * 10 + passenger1;

== matlab function Foreground/Control/Hybrid Control Code/EcoMode/Gas Pedal Scaling ==
  data: throttleIn input double; throttleOut output double
function throttleOut = fcn(throttleIn)
throttleOut=(throttleIn-16)/91;

== stateflow chart Foreground/Control/Hybrid Control Code/EcoMode/Chart ==
  state Nuetral
    during: driveTorque=0;
    during: regenTorque=0;
  state Driving
    during: driveTorque=accel;
    during: regenTorque=0;
  state RegenDrag
    during: regenTorque=dragTorque;
    during: driveTorque=0;
  state RegenBrake
    during: regenTorque=brake+dragTorque;
    during: driveTorque=0;
  (default) -> Nuetral
  Nuetral -> Driving : [accel>=accelStart]
  Driving -> RegenDrag : [accel<=accelEnd && speed>=regenStart]
  RegenDrag -> Nuetral [order 1] : [speed<=regenEnd]
  RegenBrake -> Nuetral [order 1] : [speed<=regenEnd]
  RegenDrag -> RegenBrake [order 2] : [brake>=brakeStart]
  RegenDrag -> Driving [order 3] : [accel>=accelStart]
  RegenBrake -> RegenDrag [order 2] : [brake<=brakeEnd]
  data: driveTorque output double; regenTorque output double; accel input double; brake input double; speed input double; accelStart input double; accelEnd input double; brakeStart input double; brakeEnd input double; regenStart input double; regenEnd input double; dragTorque input double

== stateflow chart Foreground/Outputs/DistributionBox/Coil1State ==
  state Coil1Disabled
    during:
    Coil1State=false;
  state Coil1Enabled
    during:
    Coil1State=true;
  (default) -> Coil1Disabled
  Coil1Disabled -> Coil1Enabled : [(TorqueRequest==0) && (BatteryVoltage>=250) && ComponentKeyed]
  Coil1Enabled -> Coil1Disabled : [(TorqueRequest==0) && !ComponentKeyed]
  data: BatteryVoltage input double; TorqueRequest input double; ComponentKeyed input boolean; Coil1State output boolean

== stateflow chart Foreground/Outputs/DistributionBox/Coil2State ==
  state Coil2Disabled
    during:
    Coil2State=false;
  state Coil2Enabled
    during:
    Coil2State=true;
  (default) -> Coil2Disabled
  Coil2Enabled -> Coil2Disabled : [!ChargerOn && !ComponentKeyed]
  Coil2Disabled -> Coil2Enabled : [!ChargerOn && ComponentKeyed]
  data: ChargerOn input boolean; ComponentKeyed input boolean; Coil2State output boolean

== stateflow chart Foreground/Outputs/DistributionBox/Coil2State1 ==
  state Coil3Disabled
    during:
    Coil3State=false;
  state Coil3Enabled
    during:
    Coil3State=true;
  (default) -> Coil3Disabled
  Coil3Disabled -> Coil3Enabled : [!HeatOn && !ACOn && ComponentKeyed]
  Coil3Enabled -> Coil3Disabled : [!HeatOn && !ACOn && !ComponentKeyed]
  data: ComponentKeyed input boolean; HeatOn input boolean; Coil3State output boolean; ACOn input boolean

== matlab function Foreground/Control/Hybrid Control Code/SUVMode/Brake Pedal Scaling ==
  data: brakeIn input double; brakeOut output double; inReverse input double
function brakeOut = fcn(brakeIn, inReverse)
if(~inReverse)
    brakeOut=1-((brakeIn-23900)/8900);
else
    brakeOut=1-((41700-brakeIn)/8900);
end
